simulink model "exampleEvaporation_Enthalpy"  (Simulink 7.6)
settings: Solver=ode45  StartTime=0.0  StopTime=10.0  RelTol=1e-3
libraries: carnot x4
settings Model: Creator=drhf  LastModifiedBy=drhf

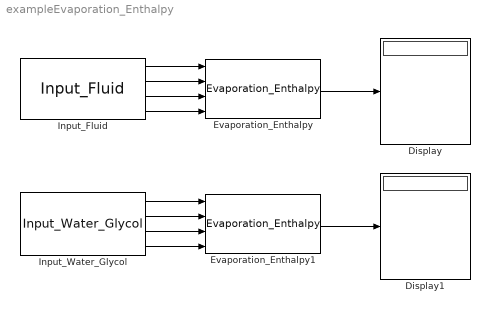
== system exampleEvaporation_Enthalpy ==
  Display : Display
  Display1 : Display
  Evaporation_Enthalpy : carnot/Basic/Material_Properties/Evaporation_Enthalpy  SystemSampleTime=-1
  Evaporation_Enthalpy1 : carnot/Basic/Material_Properties/Evaporation_Enthalpy  SystemSampleTime=-1
  Input_Fluid : carnot/Basic/Material_Properties/Input_Fluid  SystemSampleTime=-1  fluid=water  T=[10:10:50]  p=1e5  x=0.005
  Input_Water_Glycol : carnot/Basic/Material_Properties/Input_Water_Glycol  SystemSampleTime=-1  T=20  p=1e5  g=0.4
  wires:
  Input_Fluid/1 -> Evaporation_Enthalpy/1
  Input_Fluid/2 -> Evaporation_Enthalpy/2
  Input_Fluid/3 -> Evaporation_Enthalpy/3
  Input_Fluid/4 -> Evaporation_Enthalpy/4
  Evaporation_Enthalpy/1 -> Display/1
  Input_Water_Glycol/1 -> Evaporation_Enthalpy1/1
  Input_Water_Glycol/2 -> Evaporation_Enthalpy1/2
  Input_Water_Glycol/3 -> Evaporation_Enthalpy1/3
  Input_Water_Glycol/4 -> Evaporation_Enthalpy1/4
  Evaporation_Enthalpy1/1 -> Display1/1
